simulink model "w1p1"  (R2020b)
settings: Solver=VariableStepAuto  StartTime=0.0  StopTime=10  MaxStep=0.01  RelTol=1e-3
model workspace (MAT data in the model file):
  K1 = Simulink.Parameter
  K1.Value = 50
  K1.DataType = 'auto'
  K1.Dimensions = [1 1]
  K12 = Simulink.Parameter
  K12.Value = 5000
  K12.DataType = 'auto'
  K12.Dimensions = [1 1]
  M1 = Simulink.Parameter
  M1.Value = 100
  M1.DataType = 'auto'
  M1.Dimensions = [1 1]
  M2 = Simulink.Parameter
  M2.Value = 100
  M2.DataType = 'auto'
  M2.Dimensions = [1 1]
  b = Simulink.Parameter
  b.Value = 50
  b.DataType = 'auto'
  b.Dimensions = [1 1]
settings Model: Creator=Dell  LastModifiedBy=Dell

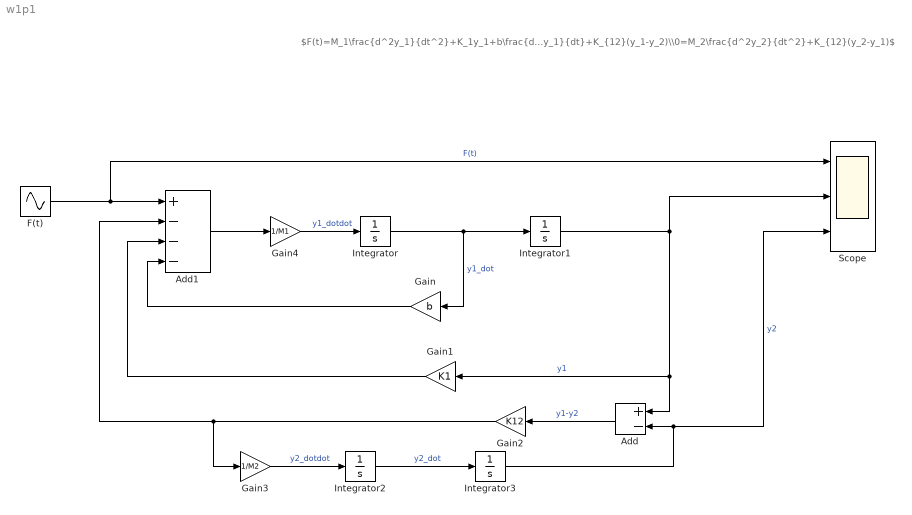
== system w1p1 ==
  note: $F(t)=M_1\frac{d^2y_1}{dt^2}+K_1y_1+b\frac{dy_1}{dt}+K_{12}(y_1-y_2)\\0=M_2\frac{d^2y_2}{dt^2}+K_{12}(y_2-y_1)$
  Add : Sum  Inputs=+-
  Add1 : Sum  Inputs=+---
  F(t) : Sin  Amplitude=2  Frequency=10  SampleTime=0
  Gain : Gain  Gain=b
  Gain1 : Gain  Gain=K1
  Gain2 : Gain  Gain=K12
  Gain3 : Gain  Gain=1/M2
  Gain4 : Gain  Gain=1/M1
  Integrator{,1..3} (4 alike) : Integrator
  Scope : Scope  NumInputPorts=3
  wires:
  Gain4/1 -> Integrator/1  "y1_dotdot"
  Integrator/1 -> Gain/1, Integrator1/1  "y1_dot"
  Integrator1/1 -> Gain1/1, Add/1, Scope/2  "y1"
  Gain3/1 -> Integrator2/1  "y2_dotdot"
  Integrator2/1 -> Integrator3/1  "y2_dot"
  Add/1 -> Gain2/1  "y1-y2"
  Gain2/1 -> Add1/2, Gain3/1
  Integrator3/1 -> Scope/3, Add/2  "y2"
  Add1/1 -> Gain4/1
  Gain/1 -> Add1/4
  Gain1/1 -> Add1/3
  F(t)/1 -> Scope/1, Add1/1  "F(t)"
